simulink model "Simulation_NoVI"  (R2022b)
settings: Solver=VariableStepAuto  StartTime=0.0  StopTime=25  RelTol=1e-3
values from neighbouring files (symbols this model uses):
  A = [0 1 1 1 ; 1 0 1 1 ; 1 1 0 1 ; 1 1 1 0]    [Primary_test1.m]    (also in init.mat = [0 1 1 1 1 0 1 1 1 1 0 1 ... (16 elements, 4x4)])
  C_f = 0.000112315*9    (= 0.001010835)    [Main.m]    (also in PSO_2paras.m = swarm(i,2); PSO_filter_2paras.m = swarm(i,2)/10000; Primary_test1.m; Script_18June.m = 0.0112315)
  f_c = 50e3    (= 50000)    [Main.m]    (also in Primary_test1.m; Script_18June.m; Script_23June.m; Script_5thJune.m)
  k = -0.5    [Main.m]    (also in Primary_test1.m; Savedata.m = 0.2909; Script_18June.m = 0.5; Script_23June.m)
  K_h11 = 0    [Main.m]    (also in PSO_HC.m = swarm(i,4); Primary_test1.m; Script_18June.m; Script_23June.m)
  K_h13 = 0    [Main.m]    (also in Primary_test1.m; Script_18June.m; Script_23June.m; Script_5thJune.m)
  K_h5 = 0    [Main.m]    (also in PSO_HC.m = swarm(i,1); Primary_test1.m = 1; Script_18June.m; Script_23June.m)
  K_h7 = 0    [Main.m]    (also in PSO_HC.m = swarm(i,2); Primary_test1.m; Script_18June.m; Script_23June.m)
  K_h9 = 0    [Main.m]    (also in PSO_HC.m = swarm(i,3); Script_18June.m; Script_23June.m; Script_5thJune.m)
  ki_pr = 160    [Main.m]    (also in PSO.m = swarm(i,2); Primary_test1.m; Savedata.m = 422.4716; Script_18June.m = 150)
  kL = 1e-7    (= 1e-07)    [Main.m]    (also in Primary_test1.m; Script_18June.m; Script_23June.m; Script_5thJune.m)
  Kp_pr = 1.7    [Main.m]    (also in PSO.m = swarm(i,1); Primary_test1.m; Savedata.m = 0.9028; Script_18June.m = 1)
  L_f = 0.000659829*1.4    (= 0.0009237606)    [Main.m]    (also in PSO_2paras.m = swarm(i,1); PSO_filter_2paras.m = swarm(i,1); Primary_test1.m; Script_18June.m = 0.000295603392)
  L_in1 = 0.35e-3    (= 0.00035)    [Main.m]    (also in Primary_test1.m; Script_18June.m; Script_23June.m; Script_5thJune.m)
  L_in2 = 0.35e-3    (= 0.00035)    [Main.m]    (also in Primary_test1.m; Script_18June.m; Script_23June.m; Script_5thJune.m)
  L_in3 = 0.35e-3    (= 0.00035)    [Main.m]    (also in Primary_test1.m; Script_18June.m; Script_23June.m; Script_5thJune.m)
  L_in4 = 0.35e-3    (= 0.00035)    [Main.m]    (also in Primary_test1.m; Script_18June.m; Script_23June.m; Script_5thJune.m)
  lambda1 = 5.5*[1 1 0.8 0.8]'    [Primary_test1.m]    (also in init.mat = [5.5 5.5 4.4 4.4])
  lambda2 = 30.5*[0.8e-2 0.8e-2 0.5e-2 0.5e-2]'    [Primary_test1.m]    (also in init.mat = [0.244 0.244 0.1525 0.1525])
  lambda3 = 62.5*[1.5e-3 1.5e-3 1e-3 1.1e-3]'    [Primary_test1.m]    (also in init.mat = [0.09375 0.09375 0.0625 0.06875])
  LD_ref1 = 100e-6    (= 0.0001)    [Main.m]    (also in Primary_test1.m; Script_18June.m = 5e-05; Script_23June.m = 1e-05; Script_5thJune.m = 1e-05)
  lo_co = 0.1    [Main.m]    (also in Primary_test1.m; Script_18June.m; Script_23June.m; Script_5thJune.m)
  load_off = 10    [Main.m]    (also in Primary_test1.m = 2; Script_18June.m = 28; Script_23June.m = 28; Script_5thJune.m)
  load_on = 0.21    [Main.m]    (also in Primary_test1.m = 1; Script_18June.m; Script_23June.m; Script_5thJune.m)
  m_p1 = 9.4e-5/droopDivide    (= 9.4e-06)    [Main.m]    (also in Primary_test1.m; Script_18June.m = 9.4e-05; Script_23June.m = 9.4e-05; Script_5thJune.m = 5e-05)
  m_p2 = 9.4e-5/droopDivide    (= 9.4e-06)    [Main.m]    (also in Primary_test1.m; Script_18June.m = 9.4e-05; Script_23June.m = 9.4e-05; Script_5thJune.m = 5e-05)
  m_p3 = 11.4e-5/droopDivide    (= 1.14e-05)    [Main.m]    (also in Primary_test1.m; Script_18June.m = 0.000114; Script_23June.m = 0.000114; Script_5thJune.m = 6.42857142857e-05)
  m_p4 = 11.4e-5/droopDivide    (= 1.14e-05)    [Main.m]    (also in Primary_test1.m; Script_18June.m = 0.000114; Script_23June.m = 0.000114; Script_5thJune.m = 6.42857142857e-05)
  N = 2    [Primary_test1.m]    (also in init.mat)
  n_q1 = 1.3e-3/droopDivide2    (= 6.5e-05)    [Main.m]    (also in Primary_test1.m; Script_18June.m; Script_23June.m; Script_5thJune.m = 0.2)
  n_q2 = 1.3e-3/droopDivide2    (= 6.5e-05)    [Main.m]    (also in Primary_test1.m; Script_18June.m; Script_23June.m; Script_5thJune.m = 0.2)
  n_q3 = 1.5e-3/droopDivide2    (= 7.5e-05)    [Main.m]    (also in Primary_test1.m; Script_18June.m; Script_23June.m; Script_5thJune.m = 0.257142857143)
  n_q4 = 1.5e-3/droopDivide2    (= 7.5e-05)    [Main.m]    (also in Primary_test1.m; Script_18June.m; Script_23June.m; Script_5thJune.m = 0.257142857143)
  Pmax = [45e3 45e3 37e3 37e3]'    [Primary_test1.m]    (also in init.mat = [45000 45000 37000 37000])
  PMW = V_nom/0.55    [Main.m]    (also in Primary_test1.m; Script_18June.m = V_nom/0.4; Script_23June.m; Script_5thJune.m = 220*sqrt(2))
  R_f = 0.35    [Main.m]    (also in PSO_filter_2paras.m = 10*L_f; Primary_test1.m; Savedata.m = 0.249593207053; Script_18June.m = 0.1)
  R_in1 = 0.03    [Main.m]    (also in Primary_test1.m; Script_18June.m; Script_23June.m; Script_5thJune.m)
  R_in2 = 0.03    [Main.m]    (also in Primary_test1.m; Script_18June.m; Script_23June.m; Script_5thJune.m)
  R_in3 = 0.03    [Main.m]    (also in Primary_test1.m; Script_18June.m; Script_23June.m; Script_5thJune.m)
  R_in4 = 0.03    [Main.m]    (also in Primary_test1.m; Script_18June.m; Script_23June.m; Script_5thJune.m)
  time_thresh = 0.2    [Main.m]    (also in Primary_test1.m; Script_18June.m; Script_23June.m; Script_5thJune.m)
  Ts = 10e-6    (= 1e-05)    [Main.m]    (also in Primary_test1.m; Script_18June.m; Script_23June.m; Script_5thJune.m)
  Tsamp = 0.1    [Primary_test1.m]    (also in init.mat)
  V_nom = 220*sqrt(2)    [Main.m]    (also in Primary_test1.m; Script_18June.m; Script_23June.m; Script_5thJune.m)
  Vdc = 600    [Main.m]    (also in Primary_test1.m; Script_18June.m; Script_23June.m; Script_5thJune.m)
  w_c_high = 2*pi*50    (= 314.159265359)    [Main.m]    (also in Primary_test1.m; Script_18June.m = 307.876080052; Script_23June.m; Script_5thJune.m = 307.876080052)
  w_nom = 2*pi*f    (= 314.159265359)    [Main.m]    (also in Primary_test1.m; Script_18June.m; Script_23June.m; Script_5thJune.m)
  wc_hc = 1    [Main.m]    (also in Primary_test1.m; Script_18June.m = 0.3; Script_23June.m; Script_5thJune.m = 0.3)
  wc_pr = 3    [Main.m]    (also in PSO.m = swarm(i,3); Primary_test1.m; Savedata.m = 1.36672; Script_18June.m = 1.5)
undefined symbols (not defined in the file or in its folder): DiscIntNeverNeededParam, i
libraries: eeGeneralControl x16, spsThreePhaseSeriesRLCBranchLib x15, spsThreePhaseVIMeasurementLib x12, spsabctoAlphaBetaZeroLib x12, spsabctodq0Lib x12, slpidlib x8, spsThreePhaseSeriesRLCLoadLib x6, spsThreePhaseBreakerLib x6, spsDCVoltageSourceLib x4, spsAlphaBetaZerotoabcLib x4, spsSeriesRLCBranchLib x4, spsTriangleGeneratorLib x4
(part 1 of 5)
settings Model: SimulationMode=accelerator  Creator=minhk  LastModifiedBy=minhk
settings SolverCC: ZeroCrossAlgorithm=Adaptive
settings DataIOCC: ReturnWorkspaceOutputs=off
settings DebuggingCC: IgnoredZcDiagnostic=none

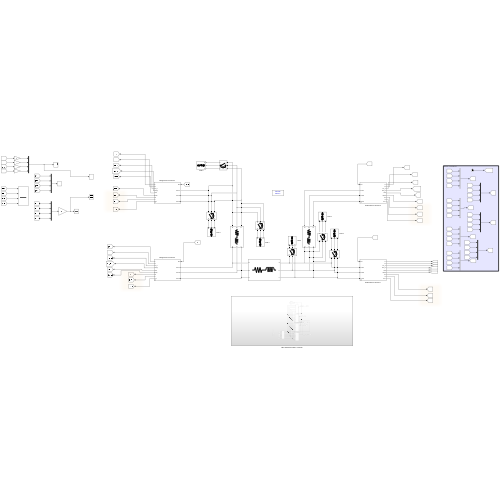
[thumbnail: Simulink's stored preview of the top-level diagram]
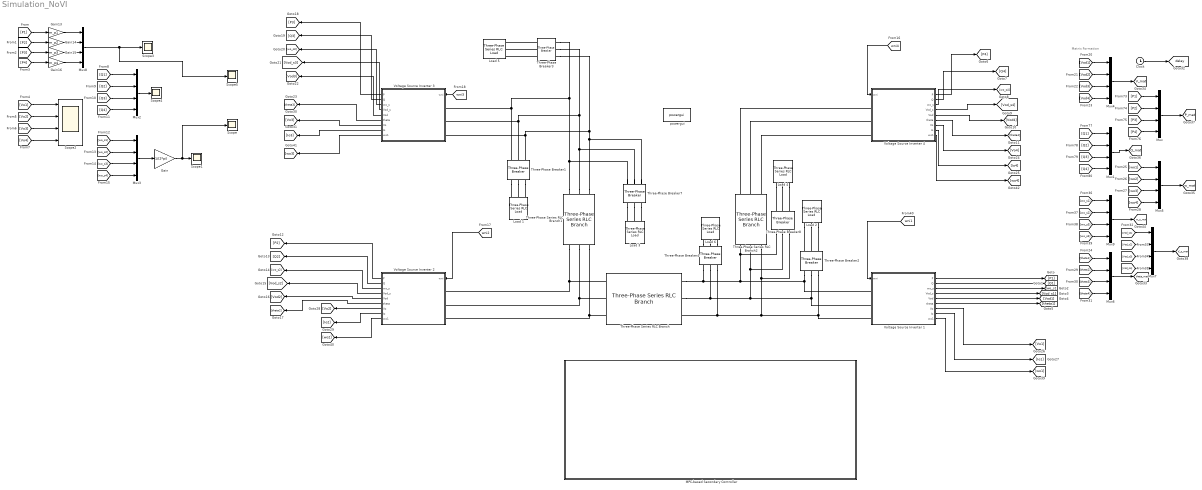
== system Simulation_NoVI ==
  note: Matrix Formation
  Clock : Clock
  Gain : Gain  Gain=1/(2*pi)
  Gain13 : Gain  Gain=m_p1
  Gain14 : Gain  Gain=m_p2
  Gain15 : Gain  Gain=m_p3
  Gain16 : Gain  Gain=m_p4
  Load 1 : spsThreePhaseSeriesRLCLoadLib/Three-Phase Series RLC Load  LConnTagsString=A|B|C  Configuration=Y (grounded)  NominalVoltage=220*sqrt(3)  Vabc=[1e3 1e3 1e3]  Vabcp=[1e3 1e3 1e3]  NominalFrequency=50  UnbalancedPower=off  ActivePower=7000*3  InductivePower=100  CapacitivePower=100  Pabc=[10e3 9e3 11e3]  QLabc=[100 90 110]  QCabc=[100 90 110]  Pabcp=[10e3 9e3 11e3]  QLabcp=[100 90 110]  QCabcp=[100 90 110]  Measurements=Branch voltages and currents  LoadType=constant Z
  Load 2 : spsThreePhaseSeriesRLCLoadLib/Three-Phase Series RLC Load  LConnTagsString=A|B|C  Configuration=Y (grounded)  NominalVoltage=220*sqrt(3)  Vabc=[1e3 1e3 1e3]  Vabcp=[1e3 1e3 1e3]  NominalFrequency=50  UnbalancedPower=off  ActivePower=7000*3  InductivePower=100  CapacitivePower=100  Pabc=[10e3 9e3 11e3]  QLabc=[100 90 110]  QCabc=[100 90 110]  Pabcp=[10e3 9e3 11e3]  QLabcp=[100 90 110]  QCabcp=[100 90 110]  Measurements=Branch voltages and currents  LoadType=constant Z
  Load 3 : spsThreePhaseSeriesRLCLoadLib/Three-Phase Series RLC Load  LConnTagsString=A|B|C  Configuration=Y (grounded)  NominalVoltage=220*sqrt(3)  Vabc=[1e3 1e3 1e3]  Vabcp=[1e3 1e3 1e3]  NominalFrequency=50  UnbalancedPower=off  ActivePower=10000*3  InductivePower=100  CapacitivePower=100  Pabc=[10e3 9e3 11e3]  QLabc=[100 90 110]  QCabc=[100 90 110]  Pabcp=[10e3 9e3 11e3]  QLabcp=[100 90 110]  QCabcp=[100 90 110]  Measurements=Branch voltages and currents  LoadType=constant Z
  Load 4 : spsThreePhaseSeriesRLCLoadLib/Three-Phase Series RLC Load  LConnTagsString=A|B|C  Configuration=Y (grounded)  NominalVoltage=220*sqrt(3)  Vabc=[1e3 1e3 1e3]  Vabcp=[1e3 1e3 1e3]  NominalFrequency=50  UnbalancedPower=off  ActivePower=10000*3  InductivePower=100  CapacitivePower=100  Pabc=[10e3 9e3 11e3]  QLabc=[100 90 110]  QCabc=[100 90 110]  Pabcp=[10e3 9e3 11e3]  QLabcp=[100 90 110]  QCabcp=[100 90 110]  Measurements=Branch voltages and currents  LoadType=constant Z
  Load 5 : spsThreePhaseSeriesRLCLoadLib/Three-Phase Series RLC Load  LConnTagsString=A|B|C  Configuration=Y (grounded)  NominalVoltage=220*sqrt(3)  Vabc=[1e3 1e3 1e3]  Vabcp=[1e3 1e3 1e3]  NominalFrequency=50  UnbalancedPower=off  ActivePower=8000*3  InductivePower=100  CapacitivePower=100  Pabc=[10e3 9e3 11e3]  QLabc=[100 90 110]  QCabc=[100 90 110]  Pabcp=[10e3 9e3 11e3]  QLabcp=[100 90 110]  QCabcp=[100 90 110]  Measurements=Branch voltages and currents  LoadType=constant Z
  Load 6 : spsThreePhaseSeriesRLCLoadLib/Three-Phase Series RLC Load  LConnTagsString=A|B|C  Configuration=Y (grounded)  NominalVoltage=220*sqrt(3)  Vabc=[1e3 1e3 1e3]  Vabcp=[1e3 1e3 1e3]  NominalFrequency=50  UnbalancedPower=off  ActivePower=7000*3  InductivePower=100  CapacitivePower=100  Pabc=[10e3 9e3 11e3]  QLabc=[100 90 110]  QCabc=[100 90 110]  Pabcp=[10e3 9e3 11e3]  QLabcp=[100 90 110]  QCabcp=[100 90 110]  Measurements=Branch voltages and currents  LoadType=constant Z
  MPC-based Secondary Controller : Subsystem
  Mux{,1..9} (10 alike) : Mux
  Scope{,1,3..5} (5 alike) : Scope
  Scope2 : Scope  NumInputPorts=4
  Three-Phase Series RLC Branch : spsThreePhaseSeriesRLCBranchLib/Three-Phase Series RLC Branch  LConnTagsString=A|B|C  RConnTagsString=A|B|C  BranchType=RL  Resistance=0.35  Inductance=1847e-6  Capacitance=1e-6  Measurements=Branch voltages and currents
  Three-Phase Series RLC Branch1 : spsThreePhaseSeriesRLCBranchLib/Three-Phase Series RLC Branch  LConnTagsString=A|B|C  RConnTagsString=A|B|C  BranchType=RL  Resistance=0.23  Inductance=318e-6  Capacitance=1e-6  Measurements=Branch voltages and currents
  Three-Phase Series RLC Branch2 : spsThreePhaseSeriesRLCBranchLib/Three-Phase Series RLC Branch  LConnTagsString=A|B|C  RConnTagsString=A|B|C  BranchType=RL  Resistance=0.23  Inductance=318e-6  Capacitance=1e-6  Measurements=Branch voltages and currents
  Three-Phase Breaker1 : spsThreePhaseBreakerLib/Three-Phase Breaker  InitialState=open  SwitchA=on  SwitchB=on  SwitchC=on  SwitchTimes=[load_on]  External=off  BreakerResistance=0.01  SnubberResistance=1e6  SnubberCapacitance=inf  Measurements=None
  Three-Phase Breaker2 : spsThreePhaseBreakerLib/Three-Phase Breaker  InitialState=open  SwitchA=on  SwitchB=on  SwitchC=on  SwitchTimes=[load_on]  External=off  BreakerResistance=0.01  SnubberResistance=1e6  SnubberCapacitance=inf  Measurements=None
  Three-Phase Breaker3 : spsThreePhaseBreakerLib/Three-Phase Breaker  InitialState=open  SwitchA=on  SwitchB=on  SwitchC=on  SwitchTimes=[load_on+13 load_off]  External=off  BreakerResistance=0.01  SnubberResistance=1e6  SnubberCapacitance=inf  Measurements=None
  Three-Phase Breaker4 : spsThreePhaseBreakerLib/Three-Phase Breaker  InitialState=open  SwitchA=on  SwitchB=on  SwitchC=on  SwitchTimes=[load_on+13 load_off]  External=off  BreakerResistance=0.01  SnubberResistance=1e6  SnubberCapacitance=inf  Measurements=None
  Three-Phase Breaker7 : spsThreePhaseBreakerLib/Three-Phase Breaker  InitialState=open  SwitchA=on  SwitchB=on  SwitchC=on  SwitchTimes=[load_on+5 ]  External=off  BreakerResistance=0.01  SnubberResistance=1e6  SnubberCapacitance=inf  Measurements=None
  Three-Phase Breaker8 : spsThreePhaseBreakerLib/Three-Phase Breaker  InitialState=open  SwitchA=on  SwitchB=on  SwitchC=on  SwitchTimes=[load_on+5]  External=off  BreakerResistance=0.01  SnubberResistance=1e6  SnubberCapacitance=inf  Measurements=None
  Voltage Source Inverter 1 : Subsystem  mask{w_nom=w_nom, V_nom=V_nom, modT=1/f_c, m_p=m_p1, n_q=n_q1, LD_ref=LD_ref1, k_LD=kL, w_c_high=[1 w_c_high], R_f=R_f, L_f=L_f, C_f=C_f, R_in=R_in2, L_in=L_in2}
      mask prompts: w_nom "Nominal frequency (radian)"; V_nom "Nominal voltage"; modT "Sampling Time"; m_p "P-w gain"; n_q "Q-V gain"; LD_ref "Reference virtual impedance (H)"; k_LD "Virtual impedance Q gain"; w_c_high "High-pass filter denominator:"; R_f "Inductor resistance:"; L_f "Filter inductance"; C_f "Filter capacitance"; R_in "Resistance coupling"; L_in "Inductance coupling"
      mask TypeOptions w_nom: w_nom/Value
      mask TypeOptions V_nom: V_nom/Value
      mask TypeOptions modT:
      | Model Predictive Control
      | /Ts
      mask TypeOptions m_p: Droop for secondary control2/Gain5/Gain
      mask TypeOptions n_q: Droop for secondary control2/Gain4/Gain
      mask TypeOptions LD_ref: LD_ref/Value
      mask TypeOptions k_LD: k_LD/Gain
      mask TypeOptions w_c_high: High-Pass Filter/Denominator
      mask TypeOptions R_f:
      | Three-Phase
      | Series RLC Branch/Resistance
      mask TypeOptions L_f:
      | Three-Phase
      | Series RLC Branch/Inductance
      mask TypeOptions C_f:
      | Three-Phase
      | Series RLC Branch2/Capacitance
      mask TypeOptions R_in:
      | Three-Phase
      | Series RLC Branch1/Resistance
      mask TypeOptions L_in:
      | Three-Phase
      | Series RLC Branch1/Inductance
      mask DialogControl ParameterGroupVar Prompt: Microgrid-wide values
      mask DialogControl Container5 Prompt: Droop value
      mask DialogControl Container8 Prompt: Filter
  Voltage Source Inverter 2 : Subsystem  mask{w_nom=w_nom, V_nom=V_nom, modT=1/f_c, m_p=m_p2, n_q=n_q2, LD_ref=LD_ref1, k_LD=kL, w_c_high=[1 w_c_high], R_f=R_f, L_f=L_f, C_f=C_f, R_in=R_in2, L_in=L_in2}
      mask prompts: w_nom "Nominal frequency (radian)"; V_nom "Nominal voltage"; modT "Sampling Time"; m_p "P-w gain"; n_q "Q-V gain"; LD_ref "Reference virtual impedance (H)"; k_LD "Virtual impedance Q gain"; w_c_high "High-pass filter denominator:"; R_f "Inductor resistance:"; L_f "Filter inductance"; C_f "Filter capacitance"; R_in "Resistance coupling"; L_in "Inductance coupling"
      mask TypeOptions w_nom: w_nom/Value
      mask TypeOptions V_nom: V_nom/Value
      mask TypeOptions modT:
      | Model Predictive Control
      | /Ts
      mask TypeOptions m_p: Droop for secondary control2/Gain5/Gain
      mask TypeOptions n_q: Droop for secondary control2/Gain4/Gain
      mask TypeOptions LD_ref: LD_ref/Value
      mask TypeOptions k_LD: k_LD/Gain
      mask TypeOptions w_c_high: High-Pass Filter/Denominator
      mask TypeOptions R_f:
      | Three-Phase
      | Series RLC Branch/Resistance
      mask TypeOptions L_f:
      | Three-Phase
      | Series RLC Branch/Inductance
      mask TypeOptions C_f:
      | Three-Phase
      | Series RLC Branch2/Capacitance
      mask TypeOptions R_in:
      | Three-Phase
      | Series RLC Branch1/Resistance
      mask TypeOptions L_in:
      | Three-Phase
      | Series RLC Branch1/Inductance
      mask DialogControl ParameterGroupVar Prompt: Microgrid-wide values
      mask DialogControl Container5 Prompt: Droop value
      mask DialogControl Container8 Prompt: Filter
  Voltage Source Inverter 3 : Subsystem  mask{w_nom=w_nom, V_nom=V_nom, modT=1/f_c, m_p=m_p3, n_q=n_q3, LD_ref=LD_ref1, k_LD=kL, w_c_high=[1 w_c_high], R_f=R_f, L_f=L_f, C_f=C_f, R_in=R_in2, L_in=L_in2}
      mask prompts: w_nom "Nominal frequency (radian)"; V_nom "Nominal voltage"; modT "Sampling Time"; m_p "P-w gain"; n_q "Q-V gain"; LD_ref "Reference virtual impedance (H)"; k_LD "Virtual impedance Q gain"; w_c_high "High-pass filter denominator:"; R_f "Inductor resistance:"; L_f "Filter inductance"; C_f "Filter capacitance"; R_in "Resistance coupling"; L_in "Inductance coupling"
      mask TypeOptions w_nom: w_nom/Value
      mask TypeOptions V_nom: V_nom/Value
      mask TypeOptions modT:
      | Model Predictive Control
      | /Ts
      mask TypeOptions m_p: Droop for secondary control2/Gain5/Gain
      mask TypeOptions n_q: Droop for secondary control2/Gain4/Gain
      mask TypeOptions LD_ref: LD_ref/Value
      mask TypeOptions k_LD: k_LD/Gain
      mask TypeOptions w_c_high: High-Pass Filter/Denominator
      mask TypeOptions R_f:
      | Three-Phase
      | Series RLC Branch/Resistance
      mask TypeOptions L_f:
      | Three-Phase
      | Series RLC Branch/Inductance
      mask TypeOptions C_f:
      | Three-Phase
      | Series RLC Branch2/Capacitance
      mask TypeOptions R_in:
      | Three-Phase
      | Series RLC Branch1/Resistance
      mask TypeOptions L_in:
      | Three-Phase
      | Series RLC Branch1/Inductance
      mask DialogControl ParameterGroupVar Prompt: Microgrid-wide values
      mask DialogControl Container5 Prompt: Droop value
      mask DialogControl Container8 Prompt: Filter
  Voltage Source Inverter 4 : Subsystem  mask{w_nom=w_nom, V_nom=V_nom, modT=1/f_c, m_p=m_p4, n_q=n_q4, LD_ref=LD_ref1, k_LD=kL, w_c_high=[1 w_c_high], R_f=R_f, L_f=L_f, C_f=C_f, R_in=R_in2, L_in=L_in2}
      mask prompts: w_nom "Nominal frequency (radian)"; V_nom "Nominal voltage"; modT "Sampling Time"; m_p "P-w gain"; n_q "Q-V gain"; LD_ref "Reference virtual impedance (H)"; k_LD "Virtual impedance Q gain"; w_c_high "High-pass filter denominator:"; R_f "Inductor resistance:"; L_f "Filter inductance"; C_f "Filter capacitance"; R_in "Resistance coupling"; L_in "Inductance coupling"
      mask TypeOptions w_nom: w_nom/Value
      mask TypeOptions V_nom: V_nom/Value
      mask TypeOptions modT:
      | Model Predictive Control
      | /Ts
      mask TypeOptions m_p: Droop for secondary control2/Gain5/Gain
      mask TypeOptions n_q: Droop for secondary control2/Gain4/Gain
      mask TypeOptions LD_ref: LD_ref/Value
      mask TypeOptions k_LD: k_LD/Gain
      mask TypeOptions w_c_high: High-Pass Filter/Denominator
      mask TypeOptions R_f:
      | Three-Phase
      | Series RLC Branch/Resistance
      mask TypeOptions L_f:
      | Three-Phase
      | Series RLC Branch/Inductance
      mask TypeOptions C_f:
      | Three-Phase
      | Series RLC Branch2/Capacitance
      mask TypeOptions R_in:
      | Three-Phase
      | Series RLC Branch1/Resistance
      mask TypeOptions L_in:
      | Three-Phase
      | Series RLC Branch1/Inductance
      mask DialogControl ParameterGroupVar Prompt: Microgrid-wide values
      mask DialogControl Container5 Prompt: Droop value
      mask DialogControl Container8 Prompt: Filter
  powergui : sps_lib/powergui  Priority=1  SimulationMode=Discrete  SampleTime=1e-4  frequency=60  Iterations=50  frequencyindice=0  Pbase=100e6  ErrMax=1e-4  UnitsV=kV  UnitsW=MW  buscounter=0  FunctionMessages=off  echomessages=off  EnableUseOfTLC=off  CurrentSourceSwitches=off  DisableSnubberDevices=off  DisableRonSwitches=off  DisableVfSwitches=off  DisplayEquations=off  AutomaticDiscreteSolvers=off  SolverType=Tustin/Backward Euler (TBE)  Interpol=off  ExternalGateDelay=off  methode=off  Ts=100  x0status=blocks  SPID=on  SwTol=0  HookPort=off  NonlinearTolerance=1e-4  nMaxIteration=100  ContinueOnMaxIteration=off  RestoreLinks=warning  ResistiveCurrentMeasurement=off  Frange=[0:2:500]  Ylog=off  Xlog=on  ShowGrid=off  save=off  variable=ZData  structure=0  ZoomFFT=off  StartTime=0.0  cycles=1  DisplayStyle=1  fundamental=60  FreqAxis=off  MaxFrequency=1000  frequencyindicesteady=1  RmsSteady=1  display=off
  tag scope: P_mat=global, Q_mat=global, V_mat=global, V_s_mat=global, delay=global, theta_mat=global, w_mat=global, w_s_mat=global
  wires:
  Voltage Source Inverter 1/1(P) -> [P1]
  Voltage Source Inverter 1/2(Q) -> [Q1]
  Voltage Source Inverter 1/3(wo_s) -> [wo_s1]
  Voltage Source Inverter 1/4(Vod_s) -> [Vod_s1]
  Voltage Source Inverter 1/5(Vod) -> [Vod1]
  Voltage Source Inverter 1/6(theta) -> [theta1]
  Voltage Source Inverter 4/1(P) -> [P4]
  Voltage Source Inverter 4/3(wo_s) -> [wo_s4]
  Voltage Source Inverter 4/2(Q) -> [Q4]
  Voltage Source Inverter 4/6(theta) -> [theta4]
  Voltage Source Inverter 4/5(Vod) -> [Vod4]
  Voltage Source Inverter 4/4(Vod_s) -> [Vod_s4]
  Voltage Source Inverter 2/1(P) -> [P2]
  Voltage Source Inverter 2/2(Q) -> [Q2]
  Voltage Source Inverter 2/3(wo_s) -> [wo_s2]
  Voltage Source Inverter 2/4(Vod_s) -> [Vod_s2]
  Voltage Source Inverter 2/5(Vod) -> [Vod2]
  Voltage Source Inverter 2/6(theta) -> [theta2]
  Voltage Source Inverter 3/6(theta) -> [theta3]
  Voltage Source Inverter 3/3(wo_s) -> [wo_s3]
  Voltage Source Inverter 3/5(Vod) -> [Vod3]
  Voltage Source Inverter 3/2(Q) -> [Q3]
  Voltage Source Inverter 3/1(P) -> [P3]
  Voltage Source Inverter 3/4(Vod_s) -> [Vod_s3]
  Voltage Source Inverter 4/7(Vo) -> [Vo4]
  Voltage Source Inverter 4/8(Io) -> [Io4]
  Voltage Source Inverter 1/8(Io) -> [Io1]
  Voltage Source Inverter 1/7(Vo) -> [Vo1]
  Voltage Source Inverter 2/7(Vo) -> [Vo2]
  Voltage Source Inverter 2/8(Io) -> [Io2]
  Voltage Source Inverter 3/7(Vo) -> [Vo3]
  Voltage Source Inverter 3/8(Io) -> [Io3]
  [Vo4] -> Scope2/4
  [Vo3] -> Scope2/3
  [Vo2] -> Scope2/2
  [Q4] -> Mux2/4
  [Q3] -> Mux2/3
  [Q1] -> Mux2/1
  [Q2] -> Mux2/2
  Mux3/1 -> Gain/1
  Gain14/1 -> Mux8/2
  [P3] -> Gain15/1
  Gain16/1 -> Mux8/4
  [P4] -> Gain16/1
  [P2] -> Gain14/1
  Gain13/1 -> Mux8/1
  [P1] -> Gain13/1
  Gain15/1 -> Mux8/3
  [Vo1] -> Scope2/1
  [wo_s2] -> Mux3/2
  [wo_s3] -> Mux3/3
  [wo_s4] -> Mux3/4
  [wo_s1] -> Mux3/1
  Mux/1 -> [P_mat]
  [Vod_s3] -> Mux7/3
  [Vod_s4] -> Mux7/4
  [Q2] -> Mux1/2
  [wo_s2] -> Mux9/2
  [P3] -> Mux/3
  [wo_s3] -> Mux9/3
  Mux9/1 -> [w_s_mat]
  Mux5/1 -> [w_mat]
  Mux7/1 -> [V_s_mat]
  Mux4/1 -> [V_mat]
  [wo_s1] -> Mux9/1
  [wo_s4] -> Mux9/4
  [Vod_s2] -> Mux7/2
  [Q4] -> Mux1/4
  Mux6/1 -> [theta_mat]
  [theta1] -> Mux6/1
  [Vod_s1] -> Mux7/1
  [wo3] -> Mux5/3
  [theta2] -> Mux6/2
  [theta3] -> Mux6/3
  [wo4] -> Mux5/4
  Clock/1 -> [delay]
  [Vod3] -> Mux4/3
  [P4] -> Mux/4
  [Vod4] -> Mux4/4
  [P1] -> Mux/1
  [wo1] -> Mux5/1
  [Q3] -> Mux1/3
  [wo2] -> Mux5/2
  [P2] -> Mux/2
  [Vod2] -> Mux4/2
  [theta4] -> Mux6/4
  [Q1] -> Mux1/1
  Mux1/1 -> [Q_mat]
  [Vod1] -> Mux4/1
  Voltage Source Inverter 1/9(wo1) -> [wo1]
  Voltage Source Inverter 4/9(wo1) -> [wo4]
  Voltage Source Inverter 3/9(wo1) -> [wo3]
  Voltage Source Inverter 2/9(wo1) -> [wo2]
  [wni1] -> Voltage Source Inverter 1/1(wni)
  [wni4] -> Voltage Source Inverter 4/1(wni)
  [wni2] -> Voltage Source Inverter 2/1(wni)
  [wni3] -> Voltage Source Inverter 3/1(wni)
  Mux2/1 -> Scope4/1
  Gain/1 -> Scope/1, Scope1/1
  Mux8/1 -> Scope5/1, Scope3/1
  connections:
  Three-Phase Series RLC Branch1/LConn1 -- Three-Phase Breaker1/RConn1 -- Voltage Source Inverter 3/LConn1 -- Three-Phase Breaker3/RConn1 -- Three-Phase Breaker7/RConn1
  Three-Phase Series RLC Branch/LConn2 -- Voltage Source Inverter 2/LConn2 -- Three-Phase Series RLC Branch1/RConn2
  Three-Phase Series RLC Branch1/LConn2 -- Three-Phase Breaker1/RConn2 -- Voltage Source Inverter 3/LConn2 -- Three-Phase Breaker3/RConn2 -- Three-Phase Breaker7/RConn2
  Three-Phase Series RLC Branch2/RConn1 -- Three-Phase Breaker2/LConn1 -- Voltage Source Inverter 1/LConn1 -- Three-Phase Breaker4/LConn1 -- Three-Phase Series RLC Branch/RConn1 -- Three-Phase Breaker8/LConn1
  Three-Phase Breaker4/LConn3 -- Three-Phase Breaker2/LConn3 -- Voltage Source Inverter 1/LConn3 -- Three-Phase Breaker8/LConn3 -- Three-Phase Series RLC Branch2/RConn3 -- Three-Phase Series RLC Branch/RConn3
  Three-Phase Series RLC Branch1/RConn1 -- Three-Phase Series RLC Branch/LConn1 -- Voltage Source Inverter 2/LConn1
  Three-Phase Series RLC Branch1/LConn3 -- Three-Phase Breaker1/RConn3 -- Voltage Source Inverter 3/LConn3 -- Three-Phase Breaker3/RConn3 -- Three-Phase Breaker7/RConn3
  Three-Phase Breaker2/LConn2 -- Three-Phase Series RLC Branch/RConn2 -- Three-Phase Breaker4/LConn2 -- Three-Phase Breaker8/LConn2 -- Three-Phase Series RLC Branch2/RConn2 -- Voltage Source Inverter 1/LConn2
  Three-Phase Series RLC Branch1/RConn3 -- Voltage Source Inverter 2/LConn3 -- Three-Phase Series RLC Branch/LConn3
  Three-Phase Series RLC Branch2/LConn1 -- Voltage Source Inverter 4/LConn1
  Three-Phase Breaker1/LConn1 -- Load 1/LConn1
  Load 6/LConn1 -- Three-Phase Breaker4/RConn1
  Three-Phase Series RLC Branch2/LConn2 -- Voltage Source Inverter 4/LConn2
  Three-Phase Breaker7/LConn3 -- Load 3/LConn3
  Load 6/LConn3 -- Three-Phase Breaker4/RConn3
  Load 6/LConn2 -- Three-Phase Breaker4/RConn2
  Three-Phase Breaker3/LConn2 -- Load 5/LConn2
  Three-Phase Breaker3/LConn3 -- Load 5/LConn3
  Three-Phase Series RLC Branch2/LConn3 -- Voltage Source Inverter 4/LConn3
  Load 2/LConn1 -- Three-Phase Breaker2/RConn1
  Three-Phase Breaker7/LConn1 -- Load 3/LConn1
  Load 4/LConn3 -- Three-Phase Breaker8/RConn3
  Load 4/LConn2 -- Three-Phase Breaker8/RConn2
  Three-Phase Breaker7/LConn2 -- Load 3/LConn2
  Load 2/LConn2 -- Three-Phase Breaker2/RConn2
  Three-Phase Breaker1/LConn3 -- Load 1/LConn3
  Three-Phase Breaker3/LConn1 -- Load 5/LConn1
  Three-Phase Breaker1/LConn2 -- Load 1/LConn2
  Load 2/LConn3 -- Three-Phase Breaker2/RConn3
  Load 4/LConn1 -- Three-Phase Breaker8/RConn1

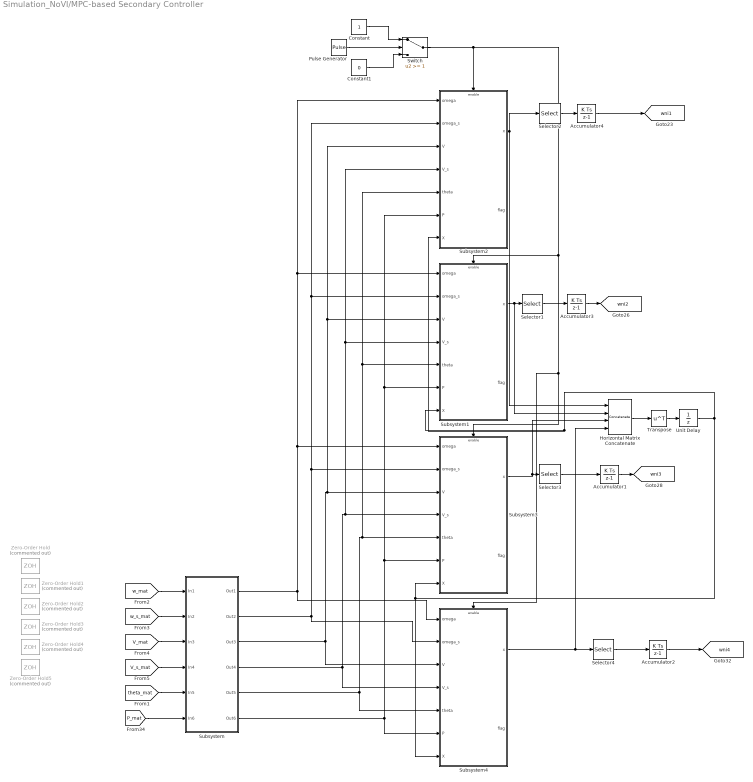
== system Simulation_NoVI/MPC-based Secondary Controller ==
  Accumulator{1..4} (4 alike) : DiscreteIntegrator  SampleTime=-1  ICPrevOutput=DiscIntNeverNeededParam  ICPrevScaledInput=DiscIntNeverNeededParam
  Constant : Constant  SampleTime=Tsamp
  Constant1 : Constant  Value=0  SampleTime=Tsamp
  Horizontal Matrix Concatenate : Concatenate  NumInputs=4  Mode=Multidimensional array  ConcatenateDimension=2
  Pulse Generator : DiscretePulseGenerator  PulseType=Time based  Period=Tsamp  PhaseDelay=time_thresh
  Selector{1..4} (4 alike) : Selector  InputPortWidth=5*N  IndexOptions=Index vector (dialog)  Indices=[N+1]  OutputSizes=1
  Subsystem : Subsystem
  Subsystem1 : Subsystem  mask{L_f=L_f, a=2, Mpw=m_p2, Tsec=Tsamp, lambda1=lambda1, lambda2=lambda2, lambda3=lambda3, Pmax=Pmax, aij=A, N=N, R_in=R_in2, L_in=L_in2}
      mask prompts: L_f "Filter Inductor"; N "Horizon"
      settings: MinAlgLoopOccurrences=on
  Subsystem2 : Subsystem  mask{L_f=L_f, a=1, Mpw=m_p1, Tsec=Tsamp, lambda1=lambda1, lambda2=lambda2, lambda3=lambda3, Pmax=Pmax, aij=A, N=N, R_in=R_in1, L_in=L_in1}
      mask prompts: L_f "Filter Inductor"; N "Horizon"
      settings: MinAlgLoopOccurrences=on
  Subsystem3 : Subsystem  mask{L_f=L_f, a=3, Mpw=m_p3, Tsec=Tsamp, lambda1=lambda1, lambda2=lambda2, lambda3=lambda3, Pmax=Pmax, aij=A, N=N, R_in=R_in3, L_in=L_in3}
      mask prompts: L_f "Filter Inductor"; N "Horizon"
      settings: MinAlgLoopOccurrences=on
  Subsystem4 : Subsystem  mask{L_f=L_f, a=4, Mpw=m_p4, Tsec=Tsamp, lambda1=lambda1, lambda2=lambda2, lambda3=lambda3, Pmax=Pmax, aij=A, N=N, R_in=R_in4, L_in=L_in4}
      mask prompts: L_f "Filter Inductor"; N "Horizon"
      settings: MinAlgLoopOccurrences=on
  Switch : Switch  Threshold=1  SaturateOnIntegerOverflow=off  InputSameDT=off
  Transpose : Math  Operator=transpose
  Unit Delay : UnitDelay  SampleTime=Tsamp*0.9  HasFrameUpgradeWarning=on
  Zero-Order Hold{,1..5} (6 alike) : ZeroOrderHold  Commented=on  SampleTime=Tsamp
  tag scope: wni1=global, wni2=global, wni3=global, wni4=global
  wires:
  Pulse Generator/1 -> Switch/2
  Constant/1 -> Switch/1
  Constant1/1 -> Switch/3
  Switch/1 -> Subsystem2/Enable, Subsystem1/Enable, Subsystem4/Enable, Subsystem3/Enable
  Subsystem2/1(x) -> Selector2/1, Horizontal Matrix Concatenate/1
  Subsystem3/1(x) -> Selector3/1, Horizontal Matrix Concatenate/3
  Horizontal Matrix Concatenate/1 -> Transpose/1
  Transpose/1 -> Unit Delay/1
  Subsystem1/1(x) -> Horizontal Matrix Concatenate/2, Selector1/1
  Subsystem4/1(x) -> Horizontal Matrix Concatenate/4, Selector4/1
  Subsystem/1(Out1) -> Subsystem4/1(omega), Subsystem3/1(omega), Subsystem1/1(omega), Subsystem2/1(omega)
  Subsystem/2(Out2) -> Subsystem4/2(omega_s), Subsystem3/2(omega_s), Subsystem1/2(omega_s), Subsystem2/2(omega_s)
  Subsystem/3(Out3) -> Subsystem4/3(V), Subsystem3/3(V), Subsystem1/3(V), Subsystem2/3(V)
  Subsystem/4(Out4) -> Subsystem4/4(V_s), Subsystem3/4(V_s), Subsystem1/4(V_s), Subsystem2/4(V_s)
  Subsystem/5(Out5) -> Subsystem4/5(theta), Subsystem3/5(theta), Subsystem1/5(theta), Subsystem2/5(theta)
  Subsystem/6(Out6) -> Subsystem4/6(P), Subsystem3/6(P), Subsystem1/6(P), Subsystem2/6(P)
  Unit Delay/1 -> Subsystem4/7(X), Subsystem3/7(X), Subsystem1/7(X), Subsystem2/7(X)
  Selector2/1 -> Accumulator4/1
  Selector1/1 -> Accumulator3/1
  Selector3/1 -> Accumulator1/1
  Selector4/1 -> Accumulator2/1
  [w_mat] -> Subsystem/1(In1)
  [w_s_mat] -> Subsystem/2(In2)
  [V_mat] -> Subsystem/3(In3)
  [V_s_mat] -> Subsystem/4(In4)
  [theta_mat] -> Subsystem/5(In5)
  [P_mat] -> Subsystem/6(In6)
  Accumulator4/1 -> [wni1]
  Accumulator3/1 -> [wni2]
  Accumulator1/1 -> [wni3]
  Accumulator2/1 -> [wni4]

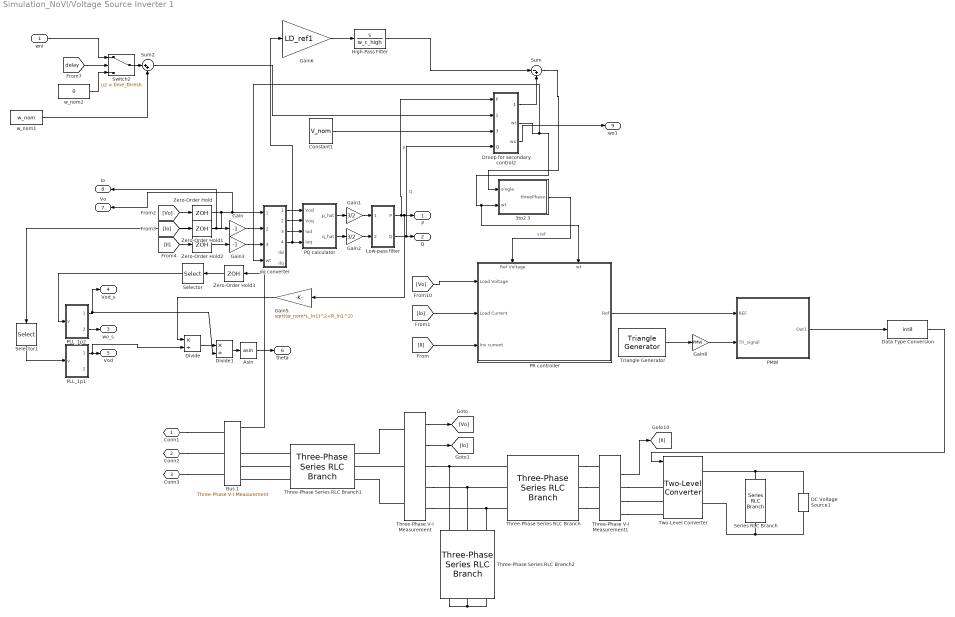
== system Simulation_NoVI/Voltage Source Inverter 1 ==
  wni : Inport
  3to2 3 : Subsystem
  Asin : Trigonometry  Operator=asin
  Bus 1 : spsThreePhaseVIMeasurementLib/Three-Phase V-I Measurement  VoltageMeasurement=phase-to-ground  SetLabelV=off  LabelV=Vbus  Vpu=off  VpuLL=off  CurrentMeasurement=yes  SetLabelI=off  LabelI=Ibus  Ipu=off  Pbase=100e6  Vbase=380  OutputType=Complex  PhasorSimulation=off  PSBequivalent=0
  Constant1 : Constant  Value=V_nom
  DC Voltage Source1 : spsDCVoltageSourceLib/DC Voltage Source  Amplitude=Vdc  Measurements=None
  Data Type Conversion : DataTypeConversion  OutDataTypeStr=int8  SaturateOnIntegerOverflow=off  RndMeth=Floor
  Divide : Product  Inputs=*/
  Divide1 : Product  Inputs=*/
  Droop for secondary control2 : Subsystem
  Gain : Gain  Gain=-1
  Gain1 : Gain  Gain=3/2
  Gain2 : Gain  Gain=3/2
  Gain3 : Gain  Gain=-1
  Gain5 : Gain  Gain=sqrt((w_nom*L_in1)^2+R_in1^2)
  Gain6 : Gain  Gain=LD_ref1
  Gain8 : Gain  Gain=PMW
  High-Pass Filter : TransferFcn  Numerator=[1 0]  Denominator=w_c_high
  Low-pass filter : Subsystem
  PLL_1p1 : Subsystem  SystemSampleTime=10*Ts
      settings: MinAlgLoopOccurrences=on
  PLL_1p2 : Subsystem  SystemSampleTime=10*Ts
      settings: MinAlgLoopOccurrences=on
  PMW : Subsystem
  PQ calculator : Subsystem
  PR controller : Subsystem
      settings: PortSchema="{\"entries\":[{\"content\":{\"sides\":[{\"content\":{\"connectorIds\":[\"In1\",\"In2\",\"In3\"]},\"type\":\"ConnectorPlacement.EquallySpacedRectSide\",\"uuid\":\"7320bc60-546b-444c-8acd-b3f08639d81a\"},{\"content\":{\"connectorIds\":[\"Out1\"],\"side\":\"RIGHT\"},\"type\":\"ConnectorPlacement.EquallySpacedRectSide\",\"uuid\":\"69cfd51f-d98e-4566-bb44-68be2b580a1e\"},{\"content\":{\"connectorIds\":[\"In4\",\"In5\"],\"side\":\"TOP\"},\"type\":\"ConnectorPlacement.EquallySpacedRectSide\",\"uuid\":\"122ed5ae-7585-404b-87e2-f9556d95c9dc\"}]},\"type\":\"ConnectorPlacement.EquallySpacedConnector\",\"uuid\":\"74384932-3814-4f3d-adae-cd0ccfea3412\"}],\"packageUris\":[\"http://schema.mathworks.com/mf0/Connector/R2020b\"],\"version\":\"1.0\"}"
  Selector : Selector  InputPortWidth=3  IndexOptions=Index vector (dialog)  Indices=[1]  OutputSizes=1
  Selector1 : Selector  InputPortWidth=3  IndexOptions=Index vector (dialog)  Indices=[1]  OutputSizes=1
  Series RLC Branch : spsSeriesRLCBranchLib/Series RLC Branch  LConnTagsString=__new0  RConnTagsString=__new0  BranchType=RC  Resistance=30  Inductance=1e-3  SetiL0=off  InitialCurrent=0  Capacitance=80e-6  Setx0=off  InitialVoltage=0  Measurements=None
  Sum : Sum  Inputs=|-+
  Sum2 : Sum  Inputs=|++
  Switch2 : Switch  Criteria=u2 > Threshold  Threshold=time_thresh  SaturateOnIntegerOverflow=off  InputSameDT=off
  Three-Phase Series RLC Branch : spsThreePhaseSeriesRLCBranchLib/Three-Phase Series RLC Branch  LConnTagsString=A|B|C  RConnTagsString=A|B|C  BranchType=RL  Resistance=R_f  Inductance=L_f  Capacitance=1e-6  Measurements=None
  Three-Phase Series RLC Branch1 : spsThreePhaseSeriesRLCBranchLib/Three-Phase Series RLC Branch  LConnTagsString=A|B|C  RConnTagsString=A|B|C  BranchType=RL  Resistance=R_in  Inductance=L_in  Capacitance=1e-6  Measurements=None
  Three-Phase Series RLC Branch2 : spsThreePhaseSeriesRLCBranchLib/Three-Phase Series RLC Branch  LConnTagsString=A|B|C  RConnTagsString=A|B|C  BranchType=C  Resistance=R_f  Inductance=1e-3  Capacitance=C_f  Measurements=None
  Three-Phase V-I Measurement : spsThreePhaseVIMeasurementLib/Three-Phase V-I Measurement  VoltageMeasurement=phase-to-ground  SetLabelV=off  LabelV=Vo1  Vpu=off  VpuLL=off  CurrentMeasurement=yes  SetLabelI=off  LabelI=Io1  Ipu=off  Pbase=100e6  Vbase=500e3  OutputType=Complex  PhasorSimulation=off  PSBequivalent=0
  Three-Phase V-I Measurement1 : spsThreePhaseVIMeasurementLib/Three-Phase V-I Measurement  VoltageMeasurement=phase-to-ground  SetLabelV=off  LabelV=Vl2  Vpu=off  VpuLL=off  CurrentMeasurement=yes  SetLabelI=off  LabelI=Il2  Ipu=off  Pbase=100e6  Vbase=500e3  OutputType=Complex  PhasorSimulation=off  PSBequivalent=0
  Triangle Generator : spsTriangleGeneratorLib/Triangle Generator  Freq=5000  Phase=90  Ts=0
  Two-Level Converter : spsTwoLevelConverterLib/Two-Level Converter  ModelType=Switching devices  Ron=1e-3  Rs=1e6  Cs=inf  Vforward=[0,0]  Ron_Diode=1e-3  Rs_Diode=1e6  Cs_Diode=inf  Vf_Diode=1e-3  Rs_CurrentSource=inf  Ron_ACsource=1e-3
  Zero-Order Hold : ZeroOrderHold  SampleTime=modT
  Zero-Order Hold1 : ZeroOrderHold  SampleTime=modT
  Zero-Order Hold2 : ZeroOrderHold  SampleTime=modT
  Zero-Order Hold3 : ZeroOrderHold  SampleTime=-1
  dq converter : Subsystem
  w_nom1 : Constant  Value=w_nom
  w_nom2 : Constant  Value=0
  Conn1 : PMIOPort  Side=Left
  Conn2 : PMIOPort  Port=2  Side=Left
  Conn3 : PMIOPort  Port=3  Side=Left
  P : Outport
  Q : Outport  Port=2
  wo_s : Outport  Port=3
  Vod_s : Outport  Port=4
  Vod : Outport  Port=5
  theta : Outport  Port=6
  Vo : Outport  Port=7
  Io : Outport  Port=8
  wo1 : Outport  Port=9
  wires:
  Three-Phase V-I Measurement/1 -> [Vo]
  Three-Phase V-I Measurement/2 -> [Io]
  Three-Phase V-I Measurement1/2 -> [Il]
  [Il] -> Zero-Order Hold2/1
  Gain1/1 -> Low-pass filter/1(p_hat)
  PQ calculator/2(q_hat) -> Gain2/1
  Gain2/1 -> Low-pass filter/2(q_hat)
  dq converter/1(Vod) -> PQ calculator/1(Vod)
  Low-pass filter/2(Q) -> Droop for secondary control2/4(Q), Q/1  "Q"
  Gain3/1 -> dq converter/3(Ildq)
  Low-pass filter/1(P) -> Droop for secondary control2/1(P), Gain5/1, P/1  "P"
  Gain/1 -> dq converter/2(Iodq)
  [Io] -> Zero-Order Hold1/1
  Zero-Order Hold2/1 -> Gain3/1
  [Vo] -> Zero-Order Hold/1
  dq converter/3(Iod) -> PQ calculator/3(Iod)
  Zero-Order Hold1/1 -> Gain/1, Io/1
  dq converter/2(Voq) -> PQ calculator/2(Voq)
  PQ calculator/1(p_hat) -> Gain1/1
  [Il] -> PR controller/3(Inv current)
  Bus 1/1 -> Zero-Order Hold3/1
  PMW/1(Out1) -> Data Type Conversion/1
  Data Type Conversion/1 -> Two-Level Converter/1
  [Io] -> PR controller/2(Load Current)
  dq converter/4(Ioq) -> Gain6/1, PQ calculator/4(Ioq)
  Gain6/1 -> High-Pass Filter/1
  Droop for secondary control2/2(wt) -> PR controller/5(wt), 3to2 3/2("wt "), dq converter/4(wt)
  Droop for secondary control2/3(wo) -> wo1/1
  [Vo] -> PR controller/1(Load Voltage)
  Constant1/1 -> Droop for secondary control2/3(V_nom)
  Sum/1 -> 3to2 3/1("single ")
  3to2 3/1(threePhase) -> PR controller/4(Ref Voltage)  "vref"
  Zero-Order Hold3/1 -> Selector/1
  Selector1/1 -> PLL_1p1/1(v)
  Selector/1 -> PLL_1p2/1(v)
  PLL_1p2/2(omega) -> wo_s/1
  Gain5/1 -> Divide/1
  Divide/1 -> Divide1/1
  PLL_1p2/1(v_dq) -> Divide1/2, Vod_s/1
  PLL_1p1/1(v_dq) -> Divide/2, Vod/1
  Divide1/1 -> Asin/1
  Asin/1 -> theta/1
  Zero-Order Hold/1 -> Selector1/1, Vo/1, dq converter/1(Vodq)
  Triangle Generator/1 -> Gain8/1
  Gain8/1 -> PMW/2(Tri_signal)
  Droop for secondary control2/1(Vref) -> Sum/2
  High-Pass Filter/1 -> Sum/1
  PR controller/1(Ref) -> PMW/1(REF)
  w_nom1/1 -> Sum2/2
  [delay] -> Switch2/2
  Switch2/1 -> Sum2/1
  wni/1 -> Switch2/1
  Sum2/1 -> Droop for secondary control2/2(w_nom)
  w_nom2/1 -> Switch2/3
  connections:
  Conn3/RConn1 -- Bus 1/LConn3
  Conn1/RConn1 -- Bus 1/LConn1
  Conn2/RConn1 -- Bus 1/LConn2
  Two-Level Converter/RConn1 -- DC Voltage Source1/RConn1 -- Series RLC Branch/LConn1
  DC Voltage Source1/LConn1 -- Two-Level Converter/RConn2 -- Series RLC Branch/RConn1
  Three-Phase V-I Measurement1/RConn1 -- Two-Level Converter/LConn1
  Three-Phase V-I Measurement1/RConn2 -- Two-Level Converter/LConn2
  Three-Phase V-I Measurement1/RConn3 -- Two-Level Converter/LConn3
  Three-Phase Series RLC Branch/RConn2 -- Three-Phase V-I Measurement1/LConn2
  Three-Phase Series RLC Branch/RConn1 -- Three-Phase V-I Measurement1/LConn1
  Three-Phase Series RLC Branch/RConn3 -- Three-Phase V-I Measurement1/LConn3
  Three-Phase Series RLC Branch2/RConn1 -- Three-Phase Series RLC Branch2/RConn3 -- Three-Phase Series RLC Branch2/RConn2
  Three-Phase V-I Measurement/RConn2 -- Three-Phase Series RLC Branch2/LConn2 -- Three-Phase Series RLC Branch/LConn2
  Three-Phase V-I Measurement/RConn1 -- Three-Phase Series RLC Branch/LConn1 -- Three-Phase Series RLC Branch2/LConn1
  Three-Phase V-I Measurement/RConn3 -- Three-Phase Series RLC Branch2/LConn3 -- Three-Phase Series RLC Branch/LConn3
  Three-Phase V-I Measurement/LConn1 -- Three-Phase Series RLC Branch1/RConn1
  Three-Phase V-I Measurement/LConn2 -- Three-Phase Series RLC Branch1/RConn2
  Three-Phase V-I Measurement/LConn3 -- Three-Phase Series RLC Branch1/RConn3
  Three-Phase Series RLC Branch1/LConn1 -- Bus 1/RConn1
  Three-Phase Series RLC Branch1/LConn2 -- Bus 1/RConn2
  Three-Phase Series RLC Branch1/LConn3 -- Bus 1/RConn3

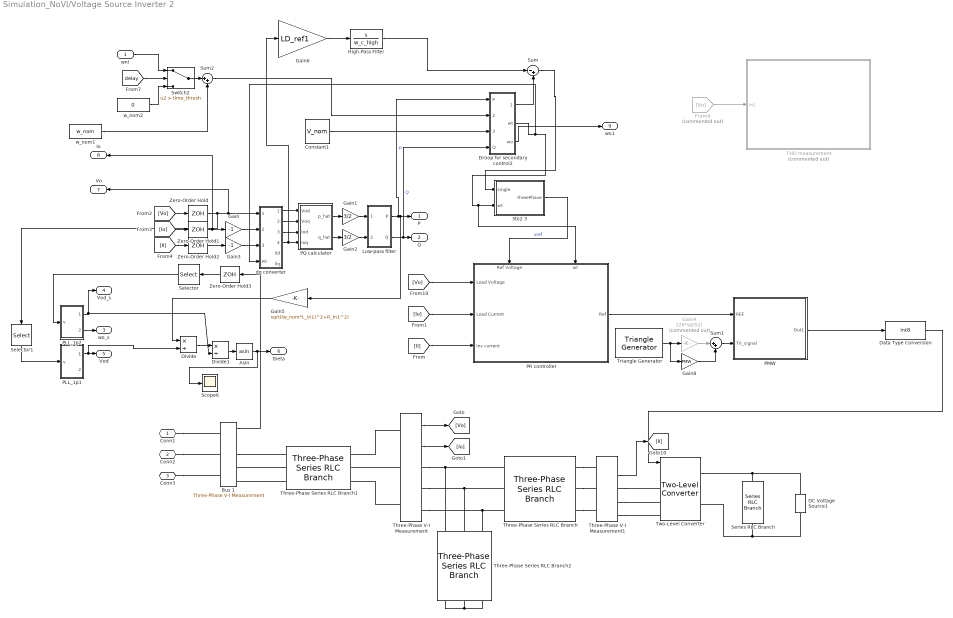
== system Simulation_NoVI/Voltage Source Inverter 2 ==
  wni : Inport
  3to2 3 : Subsystem
  Asin : Trigonometry  Operator=asin
  Bus 1 : spsThreePhaseVIMeasurementLib/Three-Phase V-I Measurement  VoltageMeasurement=phase-to-ground  SetLabelV=off  LabelV=Vbus  Vpu=off  VpuLL=off  CurrentMeasurement=yes  SetLabelI=off  LabelI=Ibus  Ipu=off  Pbase=100e6  Vbase=380  OutputType=Complex  PhasorSimulation=off  PSBequivalent=0
  Constant1 : Constant  Value=V_nom
  DC Voltage Source1 : spsDCVoltageSourceLib/DC Voltage Source  Amplitude=Vdc  Measurements=None
  Data Type Conversion : DataTypeConversion  OutDataTypeStr=int8  SaturateOnIntegerOverflow=off  RndMeth=Floor
  Divide : Product  Inputs=*/
  Divide1 : Product  Inputs=*/
  Droop for secondary control2 : Subsystem
  From9 : From  Commented=on  GotoTag=Vo
  Gain : Gain  Gain=-1
  Gain1 : Gain  Gain=3/2
  Gain2 : Gain  Gain=3/2
  Gain3 : Gain  Gain=-1
  Gain4 : Gain  Commented=on  Gain=220*sqrt(2)
  Gain5 : Gain  Gain=sqrt((w_nom*L_in1)^2+R_in1^2)
  Gain6 : Gain  Gain=LD_ref1
  Gain8 : Gain  Gain=PMW
  High-Pass Filter : TransferFcn  Numerator=[1 0]  Denominator=w_c_high
  Low-pass filter : Subsystem
  PLL_1p1 : Subsystem  SystemSampleTime=10*Ts
      settings: MinAlgLoopOccurrences=on
  PLL_1p2 : Subsystem  SystemSampleTime=10*Ts
      settings: MinAlgLoopOccurrences=on
  PMW : Subsystem
  PQ calculator : Subsystem
  PR controller : Subsystem
      settings: PortSchema="{\"entries\":[{\"content\":{\"sides\":[{\"content\":{\"connectorIds\":[\"In1\",\"In2\",\"In3\"]},\"type\":\"ConnectorPlacement.EquallySpacedRectSide\",\"uuid\":\"7320bc60-546b-444c-8acd-b3f08639d81a\"},{\"content\":{\"connectorIds\":[\"Out1\"],\"side\":\"RIGHT\"},\"type\":\"ConnectorPlacement.EquallySpacedRectSide\",\"uuid\":\"69cfd51f-d98e-4566-bb44-68be2b580a1e\"},{\"content\":{\"connectorIds\":[\"In4\",\"In5\"],\"side\":\"TOP\"},\"type\":\"ConnectorPlacement.EquallySpacedRectSide\",\"uuid\":\"122ed5ae-7585-404b-87e2-f9556d95c9dc\"}]},\"type\":\"ConnectorPlacement.EquallySpacedConnector\",\"uuid\":\"74384932-3814-4f3d-adae-cd0ccfea3412\"}],\"packageUris\":[\"http://schema.mathworks.com/mf0/Connector/R2020b\"],\"version\":\"1.0\"}"
  Scope6 : Scope
  Selector : Selector  InputPortWidth=3  IndexOptions=Index vector (dialog)  Indices=[1]  OutputSizes=1
  Selector1 : Selector  InputPortWidth=3  IndexOptions=Index vector (dialog)  Indices=[1]  OutputSizes=1
  Series RLC Branch : spsSeriesRLCBranchLib/Series RLC Branch  LConnTagsString=__new0  RConnTagsString=__new0  BranchType=RC  Resistance=30  Inductance=1e-3  SetiL0=off  InitialCurrent=0  Capacitance=80e-6  Setx0=off  InitialVoltage=0  Measurements=None
  Sum : Sum  Inputs=|-+
  Sum1 : Sum  Inputs=|++
  Sum2 : Sum  Inputs=|++
  Switch2 : Switch  Criteria=u2 > Threshold  Threshold=time_thresh  SaturateOnIntegerOverflow=off  InputSameDT=off
  THD measurement : Subsystem  Commented=on
  Three-Phase Series RLC Branch : spsThreePhaseSeriesRLCBranchLib/Three-Phase Series RLC Branch  LConnTagsString=A|B|C  RConnTagsString=A|B|C  BranchType=RL  Resistance=R_f  Inductance=L_f  Capacitance=1e-6  Measurements=None
  Three-Phase Series RLC Branch1 : spsThreePhaseSeriesRLCBranchLib/Three-Phase Series RLC Branch  LConnTagsString=A|B|C  RConnTagsString=A|B|C  BranchType=RL  Resistance=R_in  Inductance=L_in  Capacitance=1e-6  Measurements=None
  Three-Phase Series RLC Branch2 : spsThreePhaseSeriesRLCBranchLib/Three-Phase Series RLC Branch  LConnTagsString=A|B|C  RConnTagsString=A|B|C  BranchType=C  Resistance=R_f  Inductance=1e-3  Capacitance=C_f  Measurements=None
  Three-Phase V-I Measurement : spsThreePhaseVIMeasurementLib/Three-Phase V-I Measurement  VoltageMeasurement=phase-to-ground  SetLabelV=off  LabelV=Vo1  Vpu=off  VpuLL=off  CurrentMeasurement=yes  SetLabelI=off  LabelI=Io1  Ipu=off  Pbase=100e6  Vbase=500e3  OutputType=Complex  PhasorSimulation=off  PSBequivalent=0
  Three-Phase V-I Measurement1 : spsThreePhaseVIMeasurementLib/Three-Phase V-I Measurement  VoltageMeasurement=phase-to-ground  SetLabelV=off  LabelV=Vl2  Vpu=off  VpuLL=off  CurrentMeasurement=yes  SetLabelI=off  LabelI=Il2  Ipu=off  Pbase=100e6  Vbase=500e3  OutputType=Complex  PhasorSimulation=off  PSBequivalent=0
  Triangle Generator : spsTriangleGeneratorLib/Triangle Generator  Freq=5000  Phase=90  Ts=0
  Two-Level Converter : spsTwoLevelConverterLib/Two-Level Converter  ModelType=Switching devices  Ron=1e-3  Rs=1e6  Cs=inf  Vforward=[0,0]  Ron_Diode=1e-3  Rs_Diode=1e6  Cs_Diode=inf  Vf_Diode=1e-3  Rs_CurrentSource=inf  Ron_ACsource=1e-3
  Zero-Order Hold : ZeroOrderHold  SampleTime=modT
  Zero-Order Hold1 : ZeroOrderHold  SampleTime=modT
  Zero-Order Hold2 : ZeroOrderHold  SampleTime=modT
  Zero-Order Hold3 : ZeroOrderHold  SampleTime=-1
  dq converter : Subsystem
  w_nom1 : Constant  Value=w_nom
  w_nom2 : Constant  Value=0
  Conn1 : PMIOPort  Side=Left
  Conn2 : PMIOPort  Port=2  Side=Left
  Conn3 : PMIOPort  Port=3  Side=Left
  P : Outport
  Q : Outport  Port=2
  wo_s : Outport  Port=3
  Vod_s : Outport  Port=4
  Vod : Outport  Port=5
  theta : Outport  Port=6
  Vo : Outport  Port=7
  Io : Outport  Port=8
  wo1 : Outport  Port=9
  wires:
  Three-Phase V-I Measurement/1 -> [Vo]
  Three-Phase V-I Measurement/2 -> [Io]
  Three-Phase V-I Measurement1/2 -> [Il]
  [Il] -> Zero-Order Hold2/1
  Gain1/1 -> Low-pass filter/1(p_hat)
  PQ calculator/2(q_hat) -> Gain2/1
  Gain2/1 -> Low-pass filter/2(q_hat)
  dq converter/1(Vod) -> PQ calculator/1(Vod)
  Low-pass filter/2(Q) -> Droop for secondary control2/4(Q), Q/1  "Q"
  Gain3/1 -> dq converter/3(Ildq)
  Low-pass filter/1(P) -> Droop for secondary control2/1(P), Gain5/1, P/1  "P"
  Gain/1 -> dq converter/2(Iodq)
  [Io] -> Zero-Order Hold1/1
  Zero-Order Hold2/1 -> Gain3/1
  [Vo] -> Zero-Order Hold/1
  dq converter/3(Iod) -> PQ calculator/3(Iod)
  Zero-Order Hold1/1 -> Gain/1, Io/1
  dq converter/2(Voq) -> PQ calculator/2(Voq)
  PQ calculator/1(p_hat) -> Gain1/1
  [Il] -> PR controller/3(Inv current)
  Bus 1/1 -> Zero-Order Hold3/1
  PMW/1(Out1) -> Data Type Conversion/1
  Data Type Conversion/1 -> Two-Level Converter/1
  [Io] -> PR controller/2(Load Current)
  dq converter/4(Ioq) -> Gain6/1, PQ calculator/4(Ioq)
  Gain6/1 -> High-Pass Filter/1
  Droop for secondary control2/2(wt) -> PR controller/5(wt), 3to2 3/2("wt "), dq converter/4(wt)
  Droop for secondary control2/3(wo) -> wo1/1
  [Vo] -> PR controller/1(Load Voltage)
  Constant1/1 -> Droop for secondary control2/3(V_nom)
  Sum/1 -> 3to2 3/1("single ")
  3to2 3/1(threePhase) -> PR controller/4(Ref Voltage)  "vref"
  Zero-Order Hold3/1 -> Selector/1
  Selector1/1 -> PLL_1p1/1(v)
  Selector/1 -> PLL_1p2/1(v)
  PLL_1p2/2(omega) -> wo_s/1
  Gain5/1 -> Divide/1
  Divide/1 -> Divide1/1
  PLL_1p2/1(v_dq) -> Divide1/2, Vod_s/1
  PLL_1p1/1(v_dq) -> Divide/2, Vod/1
  Divide1/1 -> Asin/1
  Asin/1 -> Scope6/1, theta/1
  From9/1 -> THD measurement/1(In1)
  Zero-Order Hold/1 -> Selector1/1, Vo/1, dq converter/1(Vodq)
  Triangle Generator/1 -> Gain8/1, Gain4/1
  Gain4/1 -> Sum1/1
  Sum1/1 -> PMW/2(Tri_signal)
  Gain8/1 -> Sum1/2
  Droop for secondary control2/1(Vref) -> Sum/2
  High-Pass Filter/1 -> Sum/1
  PR controller/1(Ref) -> PMW/1(REF)
  w_nom1/1 -> Sum2/2
  [delay] -> Switch2/2
  Switch2/1 -> Sum2/1
  w_nom2/1 -> Switch2/3
  Sum2/1 -> Droop for secondary control2/2(w_nom)
  wni/1 -> Switch2/1
  connections:
  Conn3/RConn1 -- Bus 1/LConn3
  Conn1/RConn1 -- Bus 1/LConn1
  Conn2/RConn1 -- Bus 1/LConn2
  Two-Level Converter/RConn1 -- DC Voltage Source1/RConn1 -- Series RLC Branch/LConn1
  DC Voltage Source1/LConn1 -- Two-Level Converter/RConn2 -- Series RLC Branch/RConn1
  Three-Phase V-I Measurement1/RConn1 -- Two-Level Converter/LConn1
  Three-Phase V-I Measurement1/RConn2 -- Two-Level Converter/LConn2
  Three-Phase V-I Measurement1/RConn3 -- Two-Level Converter/LConn3
  Three-Phase Series RLC Branch/RConn2 -- Three-Phase V-I Measurement1/LConn2
  Three-Phase Series RLC Branch/RConn1 -- Three-Phase V-I Measurement1/LConn1
  Three-Phase Series RLC Branch/RConn3 -- Three-Phase V-I Measurement1/LConn3
  Three-Phase Series RLC Branch2/RConn1 -- Three-Phase Series RLC Branch2/RConn3 -- Three-Phase Series RLC Branch2/RConn2
  Three-Phase V-I Measurement/RConn2 -- Three-Phase Series RLC Branch2/LConn2 -- Three-Phase Series RLC Branch/LConn2
  Three-Phase V-I Measurement/RConn1 -- Three-Phase Series RLC Branch/LConn1 -- Three-Phase Series RLC Branch2/LConn1
  Three-Phase V-I Measurement/RConn3 -- Three-Phase Series RLC Branch2/LConn3 -- Three-Phase Series RLC Branch/LConn3
  Three-Phase V-I Measurement/LConn1 -- Three-Phase Series RLC Branch1/RConn1
  Three-Phase V-I Measurement/LConn2 -- Three-Phase Series RLC Branch1/RConn2
  Three-Phase V-I Measurement/LConn3 -- Three-Phase Series RLC Branch1/RConn3
  Three-Phase Series RLC Branch1/LConn1 -- Bus 1/RConn1
  Three-Phase Series RLC Branch1/LConn2 -- Bus 1/RConn2
  Three-Phase Series RLC Branch1/LConn3 -- Bus 1/RConn3
